simulink model "TypeBp"  (R2014a)
settings: Solver=ode45  StartTime=0.0  StopTime=10.0  RelTol=1e-3
values from neighbouring files (symbols this model uses):
  Act_Mat_BF = [     1,0,0,0,0,0;      0,1,0,0,0,0;      0,0,1,0,0,0;      0,0,0,1,0,0;      dv_BF,0,0,0,1,0;      0,0,0,0,0,1]    [param_PR3_noctr.m]
  Act_Mat_BR = [     1,0,0,0,0,0;      0,1,0,0,0,0;      0,0,1,0,0,0;      0,0,0,1,0,0;      dv_BR,0,0,0,1,0;      0,0,0,0,0,1]    [param_PR3_noctr.m]
  Act_Mat_IM = [     1,0,0,0,0,0;      0,1,0,0,0,0;      0,0,1,0,0,0;      0,0,0,1,0,0;      0,0,0,0,1,0;      0,0,0,0,0,1]    [param_PR3_noctr.m]
  Act_Mat_IR = [     1,0,0,0,0,0;      0,1,0,0,0,0;      0,0,1,0,0,0;      0,0,0,1,0,0;      0,0,0,0,1,0;      0,0,0,0,0,1]    [param_PR3_noctr.m]
  Act_Mat_RM = [     1,0,0,0,0,0;      0,1,0,0,0,0;      0,0,1,0,0,0;      0,0,0,1,0,0;      0,0,0,0,1,0;      0,0,0,0,0,1]    [param_PR3_noctr.m]
  Act_Mat_TM = [     1,0,0,0,0,0;      0,1,0,0,0,0;      0,0,1,0,0,0;      0,0,0,1,0,0;      0,0,0,0,1,0;      0,0,0,0,0,1]    [param_PR3_noctr.m]
  gain_act_LBF = 32.9296747504    [param_PR3_noctr.m]
  gain_act_LIM = 14.4730076835    [param_PR3_noctr.m]
  gain_act_LTM = 169.1045    [param_PR3_noctr.m]
  gain_act_PBF = 8.64557055148    [param_PR3_noctr.m]
  gain_act_PIM = 1.56040613295    [param_PR3_noctr.m]
  gain_act_PTM = 1.2097    [param_PR3_noctr.m]
  gain_act_RBF = 8.64557055148    [param_PR3_noctr.m]
  gain_act_RIM = 1.56632872419    [param_PR3_noctr.m]
  gain_act_TBF = 32.9154009359    [param_PR3_noctr.m]
  gain_act_TIM = 14.4745237388    [param_PR3_noctr.m]
  gain_act_VBF = 30.303030303    [param_PR3_noctr.m]
  gain_act_VF1 = 30.303030303    [param_PR3_noctr.m]
  gain_act_VF2 = 19.4037631453    [param_PR3_noctr.m]
  gain_act_VIM = 19.4037631453    [param_PR3_noctr.m]
  gain_act_YBF = 1.63692651118    [param_PR3_noctr.m]
  gain_act_YIM = 0.6169784052    [param_PR3_noctr.m]
  gain_act_YTM = 2.6742    [param_PR3_noctr.m]
  gain_global_LIM = 0    [param_PR3_noctr.m]
  gain_global_LTM = 0    [param_PR3_noctr.m]
  gain_LBF = 0    [param_PR3_noctr.m]
  gain_LIM = 0    [param_PR3_noctr.m]
  gain_oplev_LTM = 0    [param_PR3_noctr.m]
  gain_oplev_PIM = 0    [param_PR3_noctr.m]
  gain_oplev_PTM = 0    [param_PR3_noctr.m]
  gain_oplev_YIM = 0    [param_PR3_noctr.m]
  gain_oplev_YTM = 0    [param_PR3_noctr.m]
  gain_PBF = 0    [param_PR3_noctr.m]
  gain_PIM = 0    [param_PR3_noctr.m]
  gain_RBF = 0    [param_PR3_noctr.m]
  gain_RIM = 0    [param_PR3_noctr.m]
  gain_TBF = 0    [param_PR3_noctr.m]
  gain_TIM = 0    [param_PR3_noctr.m]
  gain_VBF = 0    [param_PR3_noctr.m]
  gain_VF1 = 0    [param_PR3_noctr.m]
  gain_VF2 = 0    [param_PR3_noctr.m]
  gain_VIM = 0    [param_PR3_noctr.m]
  gain_YBF = 0    [param_PR3_noctr.m]
  gain_YIM = 0    [param_PR3_noctr.m]
  Sens_Mat_OL = [     1,0,0,0,0,0;      0,1,0,0,0,0;      0,0,1,0,0,0;      0,0,0,1,0,0;      0,0,0,0,1,0;      0,0,0,0,0,1]    [param_PR3_noctr.m]
undefined symbols (not defined in the file or in its folder): sys1
libraries: cstblocks x21, simulink x3
settings Model: Creator=TAMA Project  LastModifiedBy=FYY
settings DataIOCC: SignalLoggingSaveFormat=ModelDataLogs
settings OptimizationCC: ExpressionDepthLimit=2147483647
settings DebuggingCC: UnderspecifiedInitializationDetection=Classic  FcnCallInpInsideContextMsg=UseLocalSettings  StateNameClashWarn=warning
settings GRTTargetCC: CombineOutputUpdateFcns=off  GRTInterface=on

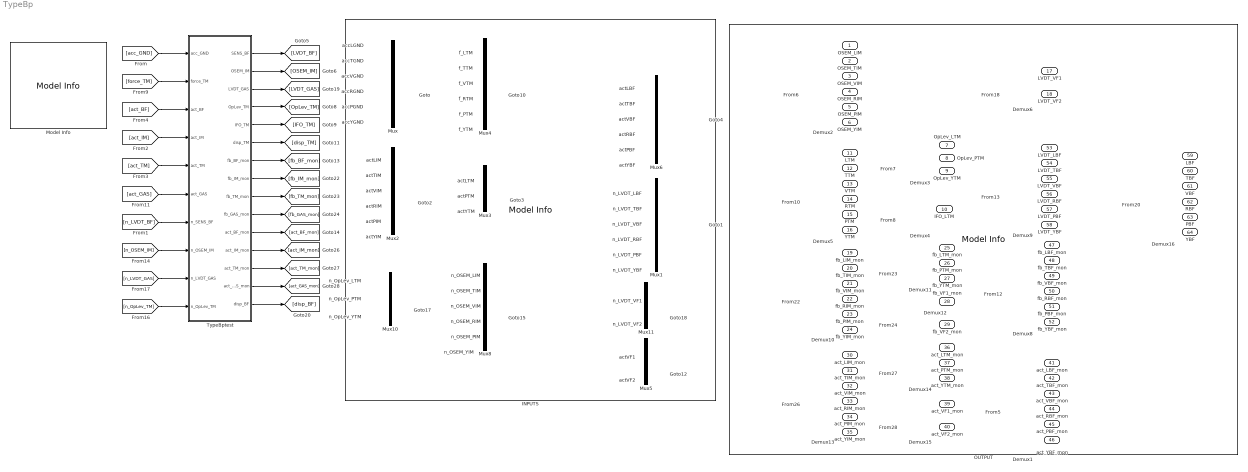
== system TypeBp ==
  accLGND : Inport
  accTGND : Inport  Port=2
  accVGND : Inport  Port=3
  accRGND : Inport  Port=4
  accPGND : Inport  Port=5
  accYGND : Inport  Port=6
  actLIM : Inport  Port=7
  actTIM : Inport  Port=8
  actVIM : Inport  Port=9
  actRIM : Inport  Port=10
  actPIM : Inport  Port=11
  actYIM : Inport  Port=12
  actLTM : Inport  Port=13
  actPTM : Inport  Port=14
  actYTM : Inport  Port=15
  f_LTM : Inport  Port=16
  f_TTM : Inport  Port=17
  f_VTM : Inport  Port=18
  f_RTM : Inport  Port=19
  f_PTM : Inport  Port=20
  f_YTM : Inport  Port=21
  actVF1 : Inport  Port=22
  actVF2 : Inport  Port=23
  n_OSEM_LIM : Inport  Port=24
  n_OSEM_TIM : Inport  Port=25
  n_OSEM_VIM : Inport  Port=26
  n_OSEM_RIM : Inport  Port=27
  n_OSEM_PIM : Inport  Port=28
  n_OSEM_YIM : Inport  Port=29
  n_OpLev_LTM : Inport  Port=30
  n_OpLev_PTM : Inport  Port=31
  n_OpLev_YTM : Inport  Port=32
  n_LVDT_VF1 : Inport  Port=33
  n_LVDT_VF2 : Inport  Port=34
  n_LVDT_LBF : Inport  Port=35
  n_LVDT_TBF : Inport  Port=36
  n_LVDT_VBF : Inport  Port=37
  n_LVDT_RBF : Inport  Port=38
  n_LVDT_PBF : Inport  Port=39
  n_LVDT_YBF : Inport  Port=40
  actLBF : Inport  Port=41
  actTBF : Inport  Port=42
  actVBF : Inport  Port=43
  actRBF : Inport  Port=44
  actPBF : Inport  Port=45
  actYBF : Inport  Port=46
  Demux{1..2,5,8..10,13,16} (8 alike) : Demux  Outputs=6
  Demux11 : Demux  Outputs=3
  Demux12 : Demux  Outputs=2
  Demux14 : Demux  Outputs=3
  Demux15 : Demux  Outputs=2
  Demux3 : Demux  Outputs=3
  Demux4 : Demux  Outputs=1
  Demux6 : Demux  Outputs=2
  INPUTS : simulink/Model-Wide Utilities/Model Info  InitialBlockCM=なし  Frame=on  DisplayStringWithTags=_  HorizontalTextAlignment=Left  LeftAlignmentValue=0.02  SourceBlockDiagram=typeBp161115simctrl_LengthOL  TagMaxNumber=20
  Model Info : simulink/Model-Wide Utilities/Model Info  InitialBlockCM=なし  Frame=on  DisplayStringWithTags=|  HorizontalTextAlignment=Left  LeftAlignmentValue=0.02  SourceBlockDiagram=typeBp161115simctrl_LengthOL  TagMaxNumber=20
      | [MODEL INFORMATION]
      | 
      | ModelName: %<ModelName>
      | LastUpdate : %<LastModificationDate>
      | 
      | TypeBp control model
  Mux{,1..2,4,6,8} (6 alike) : Mux  Inputs=6
  Mux10 : Mux  Inputs=3
  Mux11 : Mux  Inputs=2
  Mux3 : Mux  Inputs=3
  Mux5 : Mux  Inputs=2
  OUTPUT : simulink/Model-Wide Utilities/Model Info  InitialBlockCM=なし  Frame=on  DisplayStringWithTags=_  HorizontalTextAlignment=Left  LeftAlignmentValue=0.02  SourceBlockDiagram=typeBp161115simctrl_LengthOL  TagMaxNumber=20
  TypeBptest : Subsystem
  OSEM_LIM : Outport
  OSEM_TIM : Outport  Port=2
  OSEM_VIM : Outport  Port=3
  OSEM_RIM : Outport  Port=4
  OSEM_PIM : Outport  Port=5
  OSEM_YIM : Outport  Port=6
  OpLev_LTM : Outport  Port=7
  OpLev_PTM : Outport  Port=8
  OpLev_YTM : Outport  Port=9
  IFO_LTM : Outport  Port=10
  LTM : Outport  Port=11
  TTM : Outport  Port=12
  VTM : Outport  Port=13
  RTM : Outport  Port=14
  PTM : Outport  Port=15
  YTM : Outport  Port=16
  LVDT_VF1 : Outport  Port=17
  LVDT_VF2 : Outport  Port=18
  fb_LIM_mon : Outport  Port=19
  fb_TIM_mon : Outport  Port=20
  fb_VIM_mon : Outport  Port=21
  fb_RIM_mon : Outport  Port=22
  fb_PIM_mon : Outport  Port=23
  fb_YIM_mon : Outport  Port=24
  fb_LTM_mon : Outport  Port=25
  fb_PTM_mon : Outport  Port=26
  fb_YTM_mon : Outport  Port=27
  fb_VF1_mon : Outport  Port=28
  fb_VF2_mon : Outport  Port=29
  act_LIM_mon : Outport  Port=30
  act_TIM_mon : Outport  Port=31
  act_VIM_mon : Outport  Port=32
  act_RIM_mon : Outport  Port=33
  act_PIM_mon : Outport  Port=34
  act_YIM_mon : Outport  Port=35
  act_LTM_mon : Outport  Port=36
  act_PTM_mon : Outport  Port=37
  act_YTM_mon : Outport  Port=38
  act_VF1_mon : Outport  Port=39
  act_VF2_mon : Outport  Port=40
  act_LBF_mon : Outport  Port=41
  act_TBF_mon : Outport  Port=42
  act_VBF_mon : Outport  Port=43
  act_RBF_mon : Outport  Port=44
  act_PBF_mon : Outport  Port=45
  act_YBF_mon : Outport  Port=46
  fb_LBF_mon : Outport  Port=47
  fb_TBF_mon : Outport  Port=48
  fb_VBF_mon : Outport  Port=49
  fb_RBF_mon : Outport  Port=50
  fb_PBF_mon : Outport  Port=51
  fb_YBF_mon : Outport  Port=52
  LVDT_LBF : Outport  Port=53
  LVDT_TBF : Outport  Port=54
  LVDT_VBF : Outport  Port=55
  LVDT_RBF : Outport  Port=56
  LVDT_PBF : Outport  Port=57
  LVDT_YBF : Outport  Port=58
  LBF : Outport  Port=59
  TBF : Outport  Port=60
  VBF : Outport  Port=61
  RBF : Outport  Port=62
  PBF : Outport  Port=63
  YBF : Outport  Port=64
  wires:
  accLGND/1 -> Mux/1
  accTGND/1 -> Mux/2
  accVGND/1 -> Mux/3
  accRGND/1 -> Mux/4
  accPGND/1 -> Mux/5
  accYGND/1 -> Mux/6
  Mux/1 -> [acc_GND]
  actLIM/1 -> Mux2/1
  actTIM/1 -> Mux2/2
  actVIM/1 -> Mux2/3
  actRIM/1 -> Mux2/4
  actPIM/1 -> Mux2/5
  actYIM/1 -> Mux2/6
  Mux2/1 -> [act_IM]
  actLTM/1 -> Mux3/1
  actPTM/1 -> Mux3/2
  actYTM/1 -> Mux3/3
  Mux3/1 -> [act_TM]
  [OSEM_IM] -> Demux2/1
  Demux2/1 -> OSEM_LIM/1
  Demux2/2 -> OSEM_TIM/1
  Demux2/3 -> OSEM_VIM/1
  Demux2/4 -> OSEM_RIM/1
  Demux2/5 -> OSEM_PIM/1
  Demux2/6 -> OSEM_YIM/1
  [IFO_TM] -> Demux4/1
  Demux4/1 -> IFO_LTM/1
  f_LTM/1 -> Mux4/1
  f_TTM/1 -> Mux4/2
  f_VTM/1 -> Mux4/3
  Mux4/1 -> [force_TM]
  f_YTM/1 -> Mux4/6
  f_PTM/1 -> Mux4/5
  f_RTM/1 -> Mux4/4
  [disp_TM] -> Demux5/1
  Demux5/1 -> LTM/1
  Demux5/2 -> TTM/1
  Demux5/3 -> VTM/1
  Demux5/4 -> RTM/1
  Demux5/5 -> PTM/1
  Demux5/6 -> YTM/1
  actVF2/1 -> Mux5/2
  Mux5/1 -> [act_GAS]
  n_OSEM_LIM/1 -> Mux8/1
  n_OSEM_TIM/1 -> Mux8/2
  n_OSEM_VIM/1 -> Mux8/3
  n_OSEM_RIM/1 -> Mux8/4
  n_OSEM_PIM/1 -> Mux8/5
  n_OSEM_YIM/1 -> Mux8/6
  Mux8/1 -> [n_OSEM_IM]
  Mux10/1 -> [n_OpLev_TM]
  n_LVDT_VF2/1 -> Mux11/2
  Mux11/1 -> [n_LVDT_GAS]
  [LVDT_GAS] -> Demux6/1
  n_LVDT_VF1/1 -> Mux11/1
  Demux6/1 -> LVDT_VF1/1
  Demux6/2 -> LVDT_VF2/1
  actVF1/1 -> Mux5/1
  [fb_IM_mon] -> Demux10/1
  Demux10/1 -> fb_LIM_mon/1
  Demux10/2 -> fb_TIM_mon/1
  Demux10/3 -> fb_VIM_mon/1
  Demux10/4 -> fb_RIM_mon/1
  Demux10/5 -> fb_PIM_mon/1
  Demux10/6 -> fb_YIM_mon/1
  [fb_TM_mon] -> Demux11/1
  Demux11/1 -> fb_LTM_mon/1
  Demux11/2 -> fb_PTM_mon/1
  Demux11/3 -> fb_YTM_mon/1
  [fb_GAS_mon] -> Demux12/1
  Demux12/1 -> fb_VF1_mon/1
  Demux12/2 -> fb_VF2_mon/1
  [act_IM_mon] -> Demux13/1
  Demux13/1 -> act_LIM_mon/1
  Demux13/2 -> act_TIM_mon/1
  Demux13/3 -> act_VIM_mon/1
  Demux13/4 -> act_RIM_mon/1
  Demux13/5 -> act_PIM_mon/1
  Demux13/6 -> act_YIM_mon/1
  [act_TM_mon] -> Demux14/1
  Demux14/1 -> act_LTM_mon/1
  Demux14/2 -> act_PTM_mon/1
  Demux14/3 -> act_YTM_mon/1
  [act_GAS_mon] -> Demux15/1
  Demux15/1 -> act_VF1_mon/1
  Demux15/2 -> act_VF2_mon/1
  n_LVDT_TBF/1 -> Mux1/2
  Mux1/1 -> [n_LVDT_BF]
  n_LVDT_LBF/1 -> Mux1/1
  n_LVDT_VBF/1 -> Mux1/3
  actTBF/1 -> Mux6/2
  Mux6/1 -> [act_BF]
  actLBF/1 -> Mux6/1
  actVBF/1 -> Mux6/3
  [act_BF_mon] -> Demux1/1
  Demux1/1 -> act_LBF_mon/1
  Demux1/2 -> act_TBF_mon/1
  Demux1/3 -> act_VBF_mon/1
  [fb_BF_mon] -> Demux8/1
  Demux8/1 -> fb_LBF_mon/1
  Demux8/2 -> fb_TBF_mon/1
  Demux8/3 -> fb_VBF_mon/1
  [LVDT_BF] -> Demux9/1
  Demux9/1 -> LVDT_LBF/1
  Demux9/2 -> LVDT_TBF/1
  Demux9/3 -> LVDT_VBF/1
  [acc_GND] -> TypeBptest/1(acc_GND)
  [force_TM] -> TypeBptest/2(force_TM)
  [act_BF] -> TypeBptest/3(act_BF)
  [act_IM] -> TypeBptest/4(act_IM)
  [act_TM] -> TypeBptest/5(act_TM)
  [act_GAS] -> TypeBptest/6(act_GAS)
  [n_LVDT_BF] -> TypeBptest/7(n_SENS_BF)
  [n_OSEM_IM] -> TypeBptest/8(n_OSEM_IM)
  [n_LVDT_GAS] -> TypeBptest/9(n_LVDT_GAS)
  [n_OpLev_TM] -> TypeBptest/10(n_OpLev_TM)
  TypeBptest/1(SENS_BF) -> [LVDT_BF]
  TypeBptest/2(OSEM_IM) -> [OSEM_IM]
  TypeBptest/3(LVDT_GAS) -> [LVDT_GAS]
  TypeBptest/4(OpLev_TM) -> [OpLev_TM]
  TypeBptest/5(IFO_TM) -> [IFO_TM]
  TypeBptest/6(disp_TM) -> [disp_TM]
  TypeBptest/7(fb_BF_mon) -> [fb_BF_mon]
  TypeBptest/8(fb_IM_mon) -> [fb_IM_mon]
  TypeBptest/9(fb_TM_mon) -> [fb_TM_mon]
  TypeBptest/10(fb_GAS_mon) -> [fb_GAS_mon]
  TypeBptest/12(act_IM_mon) -> [act_IM_mon]
  TypeBptest/14(act_GAS_mon) -> [act_GAS_mon]
  actRBF/1 -> Mux6/4
  actPBF/1 -> Mux6/5
  actYBF/1 -> Mux6/6
  n_LVDT_RBF/1 -> Mux1/4
  n_LVDT_PBF/1 -> Mux1/5
  n_LVDT_YBF/1 -> Mux1/6
  Demux9/4 -> LVDT_RBF/1
  Demux9/5 -> LVDT_PBF/1
  Demux9/6 -> LVDT_YBF/1
  Demux8/4 -> fb_RBF_mon/1
  Demux8/5 -> fb_PBF_mon/1
  Demux8/6 -> fb_YBF_mon/1
  Demux1/4 -> act_RBF_mon/1
  Demux1/5 -> act_PBF_mon/1
  Demux1/6 -> act_YBF_mon/1
  TypeBptest/15(disp_BF) -> [disp_BF]
  [disp_BF] -> Demux16/1
  Demux16/1 -> LBF/1
  Demux16/2 -> TBF/1
  Demux16/3 -> VBF/1
  Demux16/4 -> RBF/1
  Demux16/5 -> PBF/1
  Demux16/6 -> YBF/1
  TypeBptest/11(act_BF_mon) -> [act_BF_mon]
  TypeBptest/13(act_TM_mon) -> [act_TM_mon]
  n_OpLev_PTM/1 -> Mux10/2
  n_OpLev_LTM/1 -> Mux10/1
  n_OpLev_YTM/1 -> Mux10/3
  Demux3/2 -> OpLev_PTM/1
  Demux3/3 -> OpLev_YTM/1
  Demux3/1 -> OpLev_LTM/1
  [OpLev_TM] -> Demux3/1

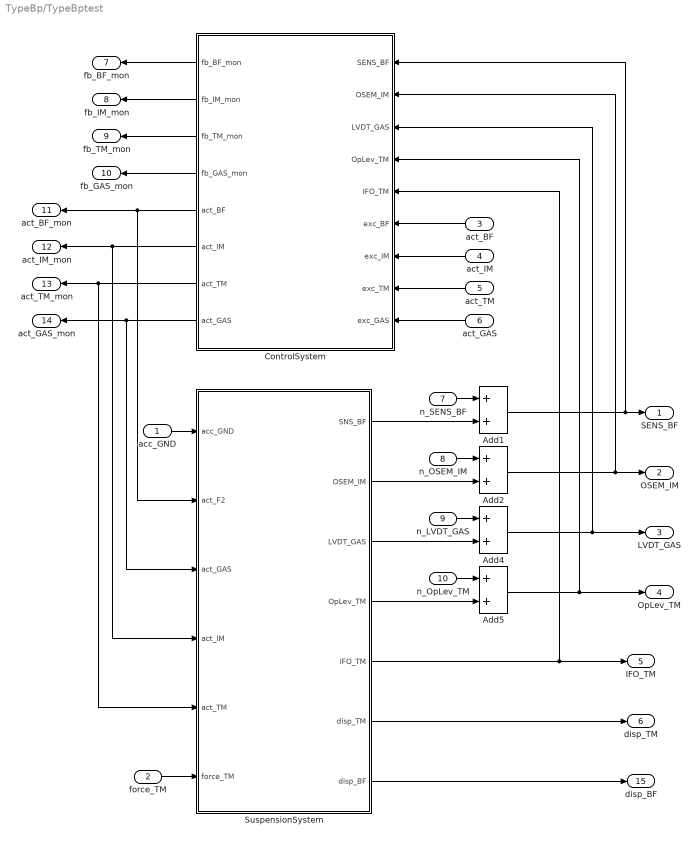
== system TypeBp/TypeBptest ==
  acc_GND : Inport
  force_TM : Inport  Port=2
  act_BF : Inport  Port=3
  act_IM : Inport  Port=4
  act_TM : Inport  Port=5
  act_GAS : Inport  Port=6
  n_SENS_BF : Inport  Port=7
  n_OSEM_IM : Inport  Port=8
  n_LVDT_GAS : Inport  Port=9
  n_OpLev_TM : Inport  Port=10
  Add{1..2,4..5} (4 alike) : Sum
  ControlSystem : Subsystem
  SuspensionSystem : Subsystem
  SENS_BF : Outport
  OSEM_IM : Outport  Port=2
  LVDT_GAS : Outport  Port=3
  OpLev_TM : Outport  Port=4
  IFO_TM : Outport  Port=5
  disp_TM : Outport  Port=6
  fb_BF_mon : Outport  Port=7
  fb_IM_mon : Outport  Port=8
  fb_TM_mon : Outport  Port=9
  fb_GAS_mon : Outport  Port=10
  act_BF_mon : Outport  Port=11
  act_IM_mon : Outport  Port=12
  act_TM_mon : Outport  Port=13
  act_GAS_mon : Outport  Port=14
  disp_BF : Outport  Port=15
  wires:
  acc_GND/1 -> SuspensionSystem/1(acc_GND)
  force_TM/1 -> SuspensionSystem/6(force_TM)
  SuspensionSystem/6(disp_TM) -> disp_TM/1
  SuspensionSystem/2(OSEM_IM) -> Add2/2
  n_OSEM_IM/1 -> Add2/1
  SuspensionSystem/5(IFO_TM) -> IFO_TM/1, ControlSystem/5(IFO_TM)
  Add2/1 -> ControlSystem/2(OSEM_IM), OSEM_IM/1
  n_LVDT_GAS/1 -> Add4/1
  SuspensionSystem/3(LVDT_GAS) -> Add4/2
  n_OpLev_TM/1 -> Add5/1
  SuspensionSystem/4(OpLev_TM) -> Add5/2
  Add4/1 -> ControlSystem/3(LVDT_GAS), LVDT_GAS/1
  Add5/1 -> ControlSystem/4(OpLev_TM), OpLev_TM/1
  Add1/1 -> ControlSystem/1(SENS_BF), SENS_BF/1
  SuspensionSystem/1(SNS_BF) -> Add1/2
  n_SENS_BF/1 -> Add1/1
  act_BF/1 -> ControlSystem/6(exc_BF)
  act_IM/1 -> ControlSystem/7(exc_IM)
  act_TM/1 -> ControlSystem/8(exc_TM)
  act_GAS/1 -> ControlSystem/9(exc_GAS)
  ControlSystem/1(fb_BF_mon) -> fb_BF_mon/1
  ControlSystem/2(fb_IM_mon) -> fb_IM_mon/1
  ControlSystem/3(fb_TM_mon) -> fb_TM_mon/1
  ControlSystem/4(fb_GAS_mon) -> fb_GAS_mon/1
  ControlSystem/5(act_BF) -> SuspensionSystem/2(act_F2), act_BF_mon/1
  ControlSystem/7(act_TM) -> SuspensionSystem/5(act_TM), act_TM_mon/1
  ControlSystem/8(act_GAS) -> SuspensionSystem/3(act_GAS), act_GAS_mon/1
  ControlSystem/6(act_IM) -> SuspensionSystem/4(act_IM), act_IM_mon/1
  SuspensionSystem/7(disp_BF) -> disp_BF/1

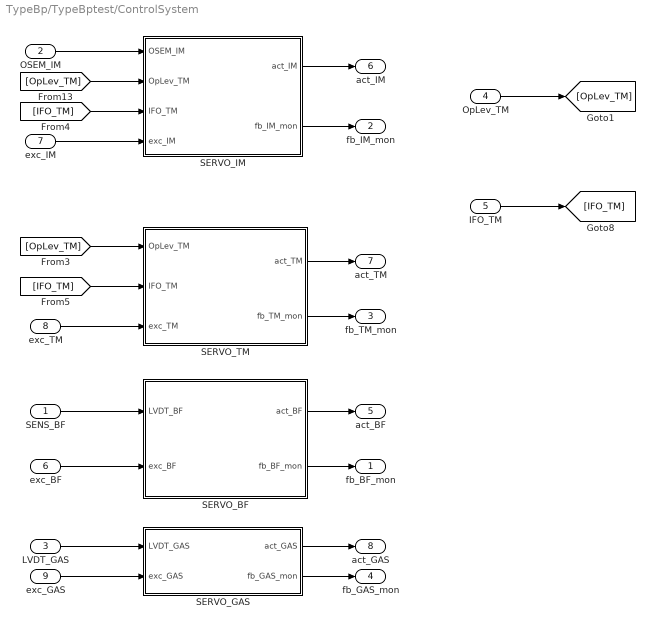
== system TypeBp/TypeBptest/ControlSystem ==
  SENS_BF : Inport
  OSEM_IM : Inport  Port=2
  LVDT_GAS : Inport  Port=3
  OpLev_TM : Inport  Port=4
  IFO_TM : Inport  Port=5
  exc_BF : Inport  Port=6
  exc_IM : Inport  Port=7
  exc_TM : Inport  Port=8
  exc_GAS : Inport  Port=9
  SERVO_BF : Subsystem
  SERVO_GAS : Subsystem
  SERVO_IM : Subsystem
  SERVO_TM : Subsystem
  fb_BF_mon : Outport
  fb_IM_mon : Outport  Port=2
  fb_TM_mon : Outport  Port=3
  fb_GAS_mon : Outport  Port=4
  act_BF : Outport  Port=5
  act_IM : Outport  Port=6
  act_TM : Outport  Port=7
  act_GAS : Outport  Port=8
  wires:
  IFO_TM/1 -> [IFO_TM]
  OpLev_TM/1 -> [OpLev_TM]
  SERVO_IM/1(act_IM) -> act_IM/1
  OSEM_IM/1 -> SERVO_IM/1(OSEM_IM)
  SERVO_TM/1(act_TM) -> act_TM/1
  [OpLev_TM] -> SERVO_IM/2(OpLev_TM)
  [OpLev_TM] -> SERVO_TM/1(OpLev_TM)
  [IFO_TM] -> SERVO_IM/3(IFO_TM)
  [IFO_TM] -> SERVO_TM/2(IFO_TM)
  exc_IM/1 -> SERVO_IM/4(exc_IM)
  exc_TM/1 -> SERVO_TM/3(exc_TM)
  SERVO_IM/2(fb_IM_mon) -> fb_IM_mon/1
  SERVO_TM/2(fb_TM_mon) -> fb_TM_mon/1
  exc_GAS/1 -> SERVO_GAS/2(exc_GAS)
  SERVO_GAS/2(fb_GAS_mon) -> fb_GAS_mon/1
  LVDT_GAS/1 -> SERVO_GAS/1(LVDT_GAS)
  SERVO_GAS/1(act_GAS) -> act_GAS/1
  SENS_BF/1 -> SERVO_BF/1(LVDT_BF)
  SERVO_BF/1(act_BF) -> act_BF/1
  exc_BF/1 -> SERVO_BF/2(exc_BF)
  SERVO_BF/2(fb_BF_mon) -> fb_BF_mon/1

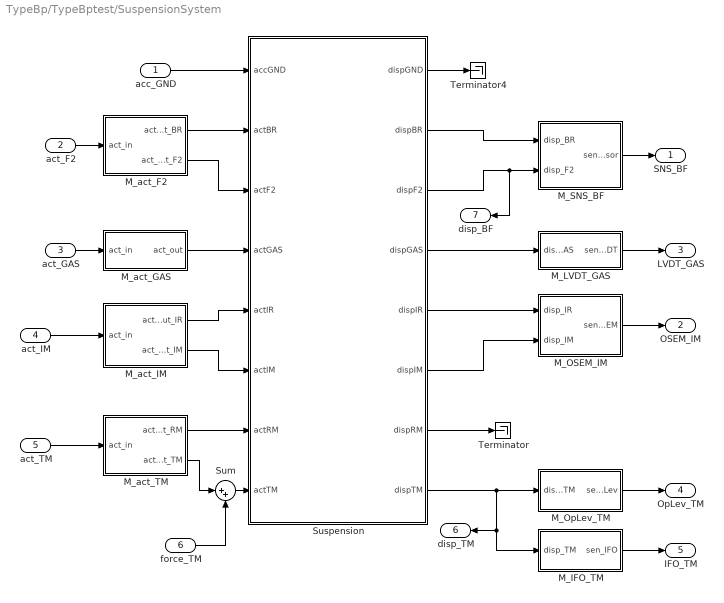
== system TypeBp/TypeBptest/SuspensionSystem ==
  acc_GND : Inport
  act_F2 : Inport  Port=2
  act_GAS : Inport  Port=3
  act_IM : Inport  Port=4
  act_TM : Inport  Port=5
  force_TM : Inport  Port=6
  M_IFO_TM : Subsystem
  M_LVDT_GAS : Subsystem
  M_OSEM_IM : Subsystem
  M_OpLev_TM : Subsystem
  M_SNS_BF : Subsystem
  M_act_F2 : Subsystem
  M_act_GAS : Subsystem
  M_act_IM : Subsystem
  M_act_TM : Subsystem
  Sum : Sum  Inputs=|++
  Suspension : Subsystem
  Terminator : Terminator
  Terminator4 : Terminator
  SNS_BF : Outport
  OSEM_IM : Outport  Port=2
  LVDT_GAS : Outport  Port=3
  OpLev_TM : Outport  Port=4
  IFO_TM : Outport  Port=5
  disp_TM : Outport  Port=6
  disp_BF : Outport  Port=7
  wires:
  act_IM/1 -> M_act_IM/1(act_in)
  act_TM/1 -> M_act_TM/1(act_in)
  act_GAS/1 -> M_act_GAS/1(act_in)
  M_OSEM_IM/1(sen_OSEM) -> OSEM_IM/1
  M_LVDT_GAS/1(sen_LVDT) -> LVDT_GAS/1
  M_IFO_TM/1(sen_IFO) -> IFO_TM/1
  M_OpLev_TM/1(sen_OpLev) -> OpLev_TM/1
  act_F2/1 -> M_act_F2/1(act_in)
  acc_GND/1 -> Suspension/1(accGND)
  M_act_F2/1(act_out_BR) -> Suspension/2(actBR)
  M_act_F2/2(act_out_F2) -> Suspension/3(actF2)
  M_act_GAS/1(act_out) -> Suspension/4(actGAS)
  M_act_IM/1(act_out_IR) -> Suspension/5(actIR)
  M_act_IM/2(act_out_IM) -> Suspension/6(actIM)
  M_act_TM/1(act_out_RM) -> Suspension/7(actRM)
  M_act_TM/2(act_out_TM) -> Sum/1
  force_TM/1 -> Sum/2
  Sum/1 -> Suspension/8(actTM)
  M_SNS_BF/1(sen_F2sensor) -> SNS_BF/1
  Suspension/2(dispBR) -> M_SNS_BF/1(disp_BR)
  Suspension/3(dispF2) -> disp_BF/1, M_SNS_BF/2(disp_F2)
  Suspension/1(dispGND) -> Terminator4/1
  Suspension/4(dispGAS) -> M_LVDT_GAS/1(disp_GAS)
  Suspension/5(dispIR) -> M_OSEM_IM/1(disp_IR)
  Suspension/6(dispIM) -> M_OSEM_IM/2(disp_IM)
  Suspension/8(dispTM) -> M_IFO_TM/1(disp_TM), disp_TM/1, M_OpLev_TM/1(disp_TM)
  Suspension/7(dispRM) -> Terminator/1

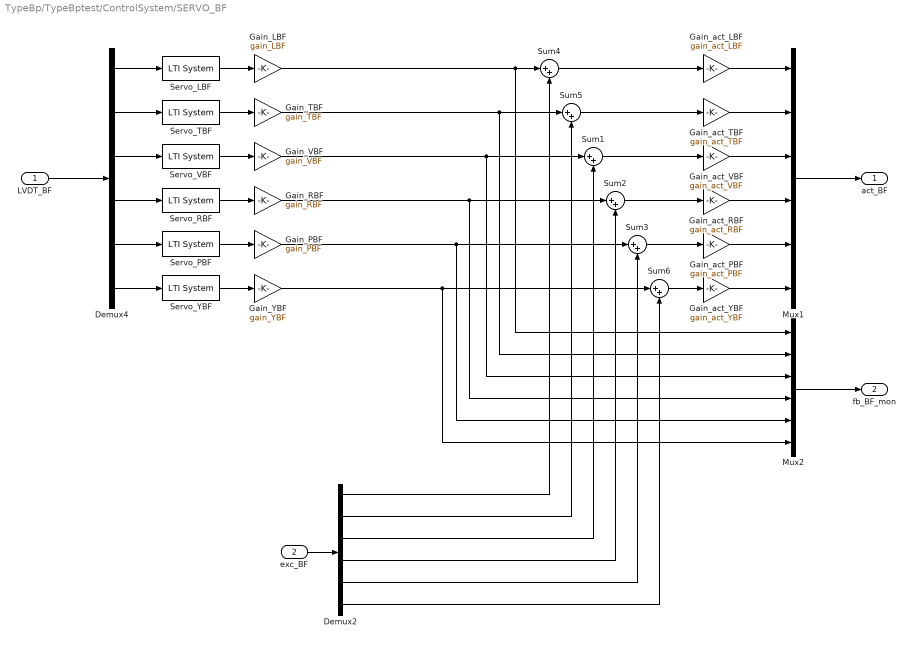
== system TypeBp/TypeBptest/ControlSystem/SERVO_BF ==
  LVDT_BF : Inport
  exc_BF : Inport  Port=2
  Demux2 : Demux  Outputs=6
  Demux4 : Demux  Outputs=6
  Gain_LBF : Gain  Gain=gain_LBF
  Gain_PBF : Gain  Gain=gain_PBF
  Gain_RBF : Gain  Gain=gain_RBF
  Gain_TBF : Gain  Gain=gain_TBF
  Gain_VBF : Gain  Gain=gain_VBF
  Gain_YBF : Gain  Gain=gain_YBF
  Gain_act_LBF : Gain  Gain=gain_act_LBF
  Gain_act_PBF : Gain  Gain=gain_act_PBF
  Gain_act_RBF : Gain  Gain=gain_act_RBF
  Gain_act_TBF : Gain  Gain=gain_act_TBF
  Gain_act_VBF : Gain  Gain=gain_act_VBF
  Gain_act_YBF : Gain  Gain=gain_act_YBF
  Mux1 : Mux  Inputs=6
  Mux2 : Mux  Inputs=6
  Servo_LBF : cstblocks/LTI System  sys=servo_LBF  IC=[]
  Servo_PBF : cstblocks/LTI System  sys=servo_PBF  IC=[]
  Servo_RBF : cstblocks/LTI System  sys=servo_RBF  IC=[]
  Servo_TBF : cstblocks/LTI System  sys=servo_TBF  IC=[]
  Servo_VBF : cstblocks/LTI System  sys=servo_VBF  IC=[]
  Servo_YBF : cstblocks/LTI System  sys=servo_YBF  IC=[]
  Sum{1..6} (6 alike) : Sum  Inputs=|++
  act_BF : Outport
  fb_BF_mon : Outport  Port=2
  wires:
  Demux4/1 -> Servo_LBF/1
  Demux4/2 -> Servo_TBF/1
  Servo_LBF/1 -> Gain_LBF/1
  Servo_TBF/1 -> Gain_TBF/1
  LVDT_BF/1 -> Demux4/1
  Mux1/1 -> act_BF/1
  Gain_act_LBF/1 -> Mux1/1
  Gain_act_TBF/1 -> Mux1/2
  Gain_LBF/1 -> Mux2/1, Sum4/1
  Sum4/1 -> Gain_act_LBF/1
  Gain_TBF/1 -> Mux2/2, Sum5/1
  Sum5/1 -> Gain_act_TBF/1
  exc_BF/1 -> Demux2/1
  Mux2/1 -> fb_BF_mon/1
  Demux4/3 -> Servo_VBF/1
  Servo_VBF/1 -> Gain_VBF/1
  Gain_act_VBF/1 -> Mux1/3
  Sum1/1 -> Gain_act_VBF/1
  Gain_VBF/1 -> Mux2/3, Sum1/1
  Demux2/1 -> Sum4/2
  Demux2/2 -> Sum5/2
  Demux2/3 -> Sum1/2
  Demux4/4 -> Servo_RBF/1
  Servo_RBF/1 -> Gain_RBF/1
  Gain_act_RBF/1 -> Mux1/4
  Gain_RBF/1 -> Mux2/4, Sum2/1
  Sum2/1 -> Gain_act_RBF/1
  Demux4/5 -> Servo_PBF/1
  Servo_PBF/1 -> Gain_PBF/1
  Gain_act_PBF/1 -> Mux1/5
  Gain_PBF/1 -> Mux2/5, Sum3/1
  Sum3/1 -> Gain_act_PBF/1
  Demux4/6 -> Servo_YBF/1
  Servo_YBF/1 -> Gain_YBF/1
  Gain_act_YBF/1 -> Mux1/6
  Gain_YBF/1 -> Mux2/6, Sum6/1
  Sum6/1 -> Gain_act_YBF/1
  Demux2/4 -> Sum2/2
  Demux2/5 -> Sum3/2
  Demux2/6 -> Sum6/2

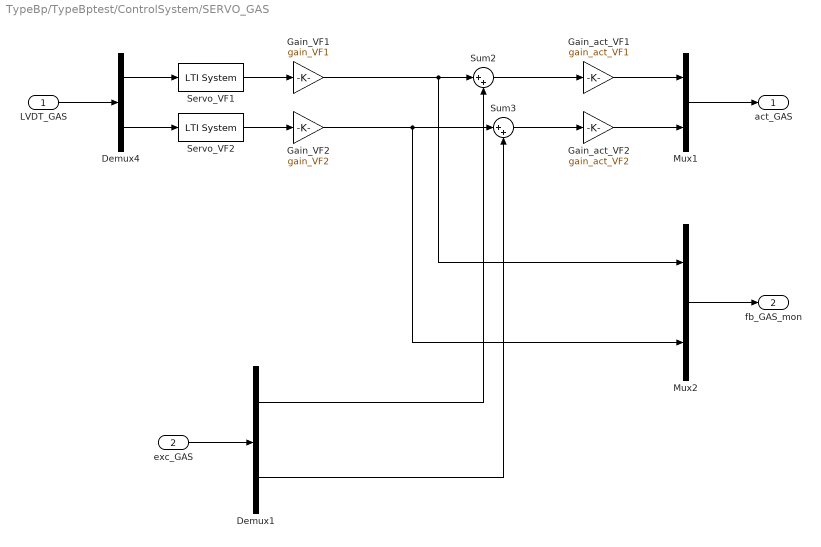
== system TypeBp/TypeBptest/ControlSystem/SERVO_GAS ==
  LVDT_GAS : Inport
  exc_GAS : Inport  Port=2
  Demux1 : Demux  Outputs=2
  Demux4 : Demux  Outputs=2
  Gain_VF1 : Gain  Gain=gain_VF1
  Gain_VF2 : Gain  Gain=gain_VF2
  Gain_act_VF1 : Gain  Gain=gain_act_VF1
  Gain_act_VF2 : Gain  Gain=gain_act_VF2
  Mux1 : Mux  Inputs=2
  Mux2 : Mux  Inputs=2
  Servo_VF1 : cstblocks/LTI System  sys=servo_VF1  IC=[]
  Servo_VF2 : cstblocks/LTI System  sys=servo_VF2  IC=[]
  Sum2 : Sum  Inputs=|++
  Sum3 : Sum  Inputs=|++
  act_GAS : Outport
  fb_GAS_mon : Outport  Port=2
  wires:
  Servo_VF1/1 -> Gain_VF1/1
  Servo_VF2/1 -> Gain_VF2/1
  LVDT_GAS/1 -> Demux4/1
  Mux1/1 -> act_GAS/1
  exc_GAS/1 -> Demux1/1
  Gain_VF1/1 -> Mux2/1, Sum2/1
  Sum2/1 -> Gain_act_VF1/1
  Gain_VF2/1 -> Mux2/2, Sum3/1
  Sum3/1 -> Gain_act_VF2/1
  Mux2/1 -> fb_GAS_mon/1
  Demux4/1 -> Servo_VF1/1
  Demux4/2 -> Servo_VF2/1
  Gain_act_VF1/1 -> Mux1/1
  Gain_act_VF2/1 -> Mux1/2
  Demux1/1 -> Sum2/2
  Demux1/2 -> Sum3/2

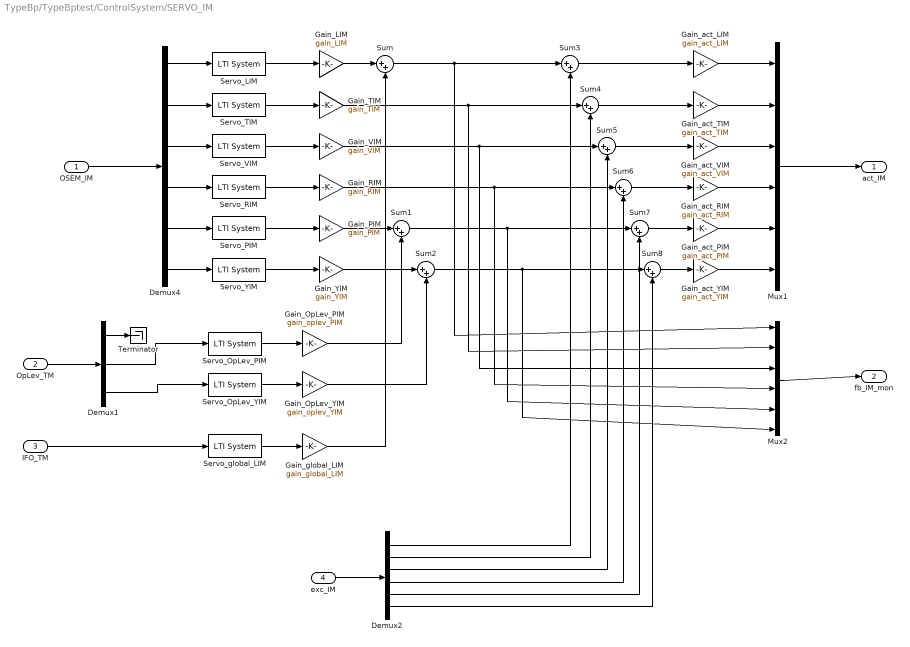
== system TypeBp/TypeBptest/ControlSystem/SERVO_IM ==
  OSEM_IM : Inport
  OpLev_TM : Inport  Port=2
  IFO_TM : Inport  Port=3
  exc_IM : Inport  Port=4
  Demux1 : Demux  Outputs=3
  Demux2 : Demux  Outputs=6
  Demux4 : Demux  Outputs=6
  Gain_LIM : Gain  Gain=gain_LIM
  Gain_OpLev_PIM : Gain  Gain=gain_oplev_PIM
  Gain_OpLev_YIM : Gain  Gain=gain_oplev_YIM
  Gain_PIM : Gain  Gain=gain_PIM
  Gain_RIM : Gain  Gain=gain_RIM
  Gain_TIM : Gain  Gain=gain_TIM
  Gain_VIM : Gain  Gain=gain_VIM
  Gain_YIM : Gain  Gain=gain_YIM
  Gain_act_LIM : Gain  Gain=gain_act_LIM
  Gain_act_PIM : Gain  Gain=gain_act_PIM
  Gain_act_RIM : Gain  Gain=gain_act_RIM
  Gain_act_TIM : Gain  Gain=gain_act_TIM
  Gain_act_VIM : Gain  Gain=gain_act_VIM
  Gain_act_YIM : Gain  Gain=gain_act_YIM
  Gain_global_LIM : Gain  Gain=gain_global_LIM
  Mux1 : Mux  Inputs=6
  Mux2 : Mux  Inputs=6
  Servo_LIM : cstblocks/LTI System  sys=servo_LIM  IC=[]
  Servo_OpLev_PIM : cstblocks/LTI System  sys=servo_oplev_PIM  IC=[]
  Servo_OpLev_YIM : cstblocks/LTI System  sys=servo_oplev_YIM  IC=[]
  Servo_PIM : cstblocks/LTI System  sys=servo_PIM  IC=[]
  Servo_RIM : cstblocks/LTI System  sys=servo_RIM  IC=[]
  Servo_TIM : cstblocks/LTI System  sys=servo_TIM  IC=[]
  Servo_VIM : cstblocks/LTI System  sys=servo_VIM  IC=[]
  Servo_YIM : cstblocks/LTI System  sys=servo_YIM  IC=[]
  Servo_global_LIM : cstblocks/LTI System  sys=servo_global_LIM  IC=[]
  Sum{,1..8} (9 alike) : Sum  Inputs=|++
  Terminator : Terminator
  act_IM : Outport
  fb_IM_mon : Outport  Port=2
  wires:
  Demux4/1 -> Servo_LIM/1
  Demux4/2 -> Servo_TIM/1
  Demux4/3 -> Servo_VIM/1
  Servo_LIM/1 -> Gain_LIM/1
  Servo_TIM/1 -> Gain_TIM/1
  Servo_VIM/1 -> Gain_VIM/1
  Mux1/1 -> act_IM/1
  Gain_act_LIM/1 -> Mux1/1
  Gain_act_TIM/1 -> Mux1/2
  Gain_act_VIM/1 -> Mux1/3
  OSEM_IM/1 -> Demux4/1
  Servo_RIM/1 -> Gain_RIM/1
  Servo_PIM/1 -> Gain_PIM/1
  Servo_YIM/1 -> Gain_YIM/1
  Demux4/4 -> Servo_RIM/1
  Demux4/5 -> Servo_PIM/1
  Demux4/6 -> Servo_YIM/1
  Gain_act_RIM/1 -> Mux1/4
  Gain_act_PIM/1 -> Mux1/5
  Gain_act_YIM/1 -> Mux1/6
  OpLev_TM/1 -> Demux1/1
  IFO_TM/1 -> Servo_global_LIM/1
  Gain_LIM/1 -> Sum/1
  Servo_global_LIM/1 -> Gain_global_LIM/1
  Gain_PIM/1 -> Sum1/1
  Gain_YIM/1 -> Sum2/1
  Gain_global_LIM/1 -> Sum/2
  Servo_OpLev_PIM/1 -> Gain_OpLev_PIM/1
  Servo_OpLev_YIM/1 -> Gain_OpLev_YIM/1
  Gain_OpLev_PIM/1 -> Sum1/2
  Gain_OpLev_YIM/1 -> Sum2/2
  Sum/1 -> Sum3/1, Mux2/1
  Sum3/1 -> Gain_act_LIM/1
  Gain_TIM/1 -> Mux2/2, Sum4/1
  Sum4/1 -> Gain_act_TIM/1
  Gain_VIM/1 -> Mux2/3, Sum5/1
  Sum5/1 -> Gain_act_VIM/1
  Gain_RIM/1 -> Sum6/1, Mux2/4
  Sum6/1 -> Gain_act_RIM/1
  Sum1/1 -> Sum7/1, Mux2/5
  Sum7/1 -> Gain_act_PIM/1
  Sum2/1 -> Sum8/1, Mux2/6
  Sum8/1 -> Gain_act_YIM/1
  Demux2/1 -> Sum3/2
  Demux2/2 -> Sum4/2
  Demux2/3 -> Sum5/2
  Demux2/4 -> Sum6/2
  Demux2/5 -> Sum7/2
  Demux2/6 -> Sum8/2
  exc_IM/1 -> Demux2/1
  Mux2/1 -> fb_IM_mon/1
  Demux1/2 -> Servo_OpLev_PIM/1
  Demux1/3 -> Servo_OpLev_YIM/1
  Demux1/1 -> Terminator/1

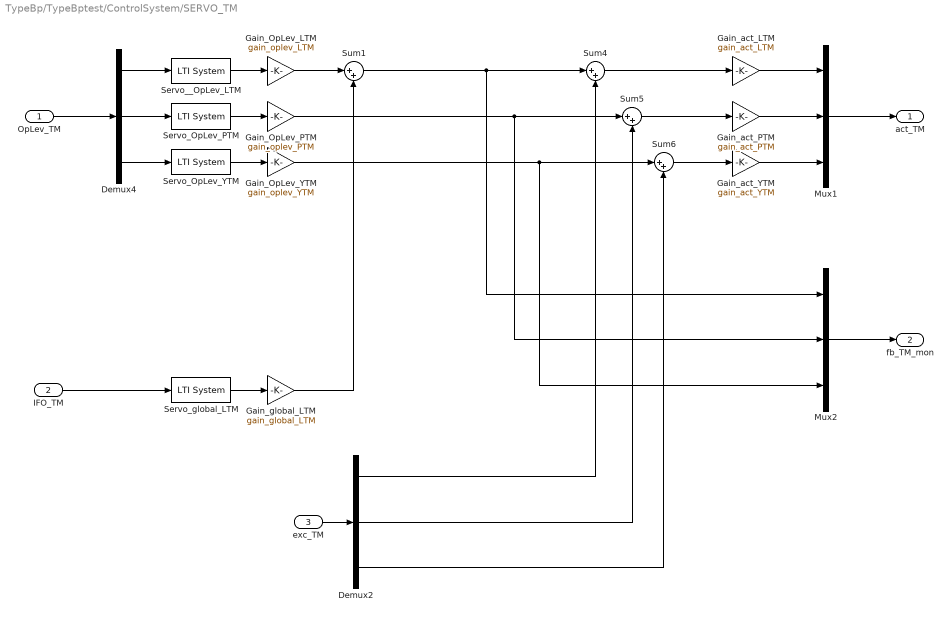
== system TypeBp/TypeBptest/ControlSystem/SERVO_TM ==
  OpLev_TM : Inport
  IFO_TM : Inport  Port=2
  exc_TM : Inport  Port=3
  Demux2 : Demux  Outputs=3
  Demux4 : Demux  Outputs=3
  Gain_OpLev_LTM : Gain  Gain=gain_oplev_LTM
  Gain_OpLev_PTM : Gain  Gain=gain_oplev_PTM
  Gain_OpLev_YTM : Gain  Gain=gain_oplev_YTM
  Gain_act_LTM : Gain  Gain=gain_act_LTM
  Gain_act_PTM : Gain  Gain=gain_act_PTM
  Gain_act_YTM : Gain  Gain=gain_act_YTM
  Gain_global_LTM : Gain  Gain=gain_global_LTM
  Mux1 : Mux  Inputs=3
  Mux2 : Mux  Inputs=3
  Servo_OpLev_PTM : cstblocks/LTI System  sys=servo_oplev_PTM  IC=[]
  Servo_OpLev_YTM : cstblocks/LTI System  sys=servo_oplev_YTM  IC=[]
  Servo__OpLev_LTM : cstblocks/LTI System  sys=servo_oplev_LTM  IC=[]
  Servo_global_LTM : cstblocks/LTI System  sys=servo_global_LTM  IC=[]
  Sum{1,4..6} (4 alike) : Sum  Inputs=|++
  act_TM : Outport
  fb_TM_mon : Outport  Port=2
  wires:
  Demux4/1 -> Servo__OpLev_LTM/1
  Demux4/2 -> Servo_OpLev_PTM/1
  Demux4/3 -> Servo_OpLev_YTM/1
  Servo__OpLev_LTM/1 -> Gain_OpLev_LTM/1
  Servo_OpLev_PTM/1 -> Gain_OpLev_PTM/1
  Servo_OpLev_YTM/1 -> Gain_OpLev_YTM/1
  OpLev_TM/1 -> Demux4/1
  Mux1/1 -> act_TM/1
  IFO_TM/1 -> Servo_global_LTM/1
  Servo_global_LTM/1 -> Gain_global_LTM/1
  Gain_OpLev_LTM/1 -> Sum1/1
  Gain_global_LTM/1 -> Sum1/2
  Gain_act_LTM/1 -> Mux1/1
  Gain_act_PTM/1 -> Mux1/2
  Gain_act_YTM/1 -> Mux1/3
  Sum1/1 -> Mux2/1, Sum4/1
  Sum4/1 -> Gain_act_LTM/1
  Gain_OpLev_PTM/1 -> Mux2/2, Sum5/1
  Sum5/1 -> Gain_act_PTM/1
  Gain_OpLev_YTM/1 -> Mux2/3, Sum6/1
  Sum6/1 -> Gain_act_YTM/1
  exc_TM/1 -> Demux2/1
  Demux2/1 -> Sum4/2
  Demux2/2 -> Sum5/2
  Demux2/3 -> Sum6/2
  Mux2/1 -> fb_TM_mon/1

== system TypeBp/TypeBptest/SuspensionSystem/M_IFO_TM ==
  disp_TM : Inport
  Add2 : Sum  Inputs=++++
  Demux4 : Demux  Outputs=6
  Gain1 : Gain  Gain=1/300
  Gain2 : Gain  Gain=1e-3
  Gain3 : Gain  Gain=1e-3
  Terminator1 : Terminator
  Terminator3 : Terminator
  sen_IFO : Outport
  wires:
  disp_TM/1 -> Demux4/1
  Demux4/4 -> Terminator3/1
  Demux4/3 -> Gain1/1
  Demux4/2 -> Terminator1/1
  Add2/1 -> sen_IFO/1
  Demux4/1 -> Add2/1
  Gain1/1 -> Add2/2
  Demux4/5 -> Gain2/1
  Gain3/1 -> Add2/4
  Gain2/1 -> Add2/3
  Demux4/6 -> Gain3/1

== system TypeBp/TypeBptest/SuspensionSystem/M_LVDT_GAS ==
  disp_GAS : Inport
  Add1 : Sum  Inputs=-+
  Add2 : Sum  Inputs=-+
  Demux4 : Demux  Outputs=3
  Mux3 : Mux  Inputs=2
  sen_LVDT : Outport
  wires:
  disp_GAS/1 -> Demux4/1
  Demux4/1 -> Add2/1
  Demux4/2 -> Add1/1, Add2/2
  Demux4/3 -> Add1/2
  Add2/1 -> Mux3/1
  Add1/1 -> Mux3/2
  Mux3/1 -> sen_LVDT/1

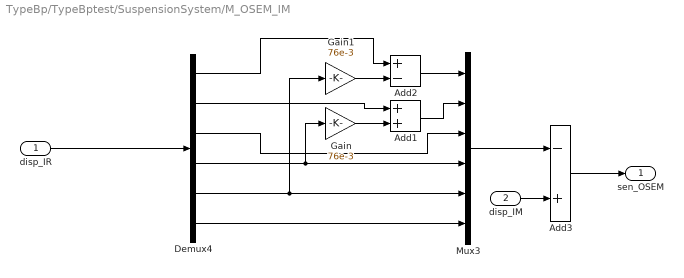
== system TypeBp/TypeBptest/SuspensionSystem/M_OSEM_IM ==
  disp_IR : Inport
  disp_IM : Inport  Port=2
  Add1 : Sum
  Add2 : Sum  Inputs=+-
  Add3 : Sum  Inputs=-+
  Demux4 : Demux  Outputs=6
  Gain : Gain  Gain=76e-3
  Gain1 : Gain  Gain=76e-3
  Mux3 : Mux  Inputs=6
  sen_OSEM : Outport
  wires:
  disp_IM/1 -> Add3/2
  disp_IR/1 -> Demux4/1
  Demux4/6 -> Mux3/6
  Mux3/1 -> Add3/1
  Add3/1 -> sen_OSEM/1
  Demux4/1 -> Add2/1
  Demux4/2 -> Add1/1
  Demux4/3 -> Mux3/3
  Demux4/4 -> Gain/1, Mux3/4
  Demux4/5 -> Gain1/1, Mux3/5
  Gain1/1 -> Add2/2
  Gain/1 -> Add1/2
  Add1/1 -> Mux3/2
  Add2/1 -> Mux3/1

== system TypeBp/TypeBptest/SuspensionSystem/M_OpLev_TM ==
  disp_TM : Inport
  Demux1 : Demux  Outputs=6
  Mux1 : Mux  Inputs=3
  Sens_Mat_OL : Constant  Value=Sens_Mat_OL  VectorParams1D=off
  TM_OpLev_coupling : Product  Multiplication=Matrix(*)
  Terminator4 : Terminator
  Terminator5 : Terminator
  Terminator6 : Terminator
  sen_OpLev : Outport
  wires:
  Demux1/5 -> Mux1/2
  Demux1/6 -> Mux1/3
  Demux1/4 -> Terminator6/1
  Demux1/3 -> Terminator5/1
  Demux1/2 -> Terminator4/1
  Demux1/1 -> Mux1/1
  Mux1/1 -> sen_OpLev/1
  TM_OpLev_coupling/1 -> Demux1/1
  Sens_Mat_OL/1 -> TM_OpLev_coupling/1
  disp_TM/1 -> TM_OpLev_coupling/2

== system TypeBp/TypeBptest/SuspensionSystem/M_SNS_BF ==
  disp_BR : Inport
  disp_F2 : Inport  Port=2
  Add2 : Sum  Inputs=-+
  sen_F2sensor : Outport
  wires:
  Add2/1 -> sen_F2sensor/1
  disp_BR/1 -> Add2/1
  disp_F2/1 -> Add2/2

== system TypeBp/TypeBptest/SuspensionSystem/M_act_F2 ==
  act_in : Inport
  Act_Mat_BF : Constant  Value=Act_Mat_BF  VectorParams1D=off
  Act_Mat_BR : Constant  Value=Act_Mat_BR  VectorParams1D=off
  BF_coupling : Product  Multiplication=Matrix(*)
  BR_coupling : Product  Multiplication=Matrix(*)
  Gain2 : Gain  Gain=-1
  act_out_BR : Outport
  act_out_F2 : Outport  Port=2
  wires:
  act_in/1 -> BF_coupling/2, Gain2/1
  Gain2/1 -> BR_coupling/2
  Act_Mat_BR/1 -> BR_coupling/1
  BR_coupling/1 -> act_out_BR/1
  Act_Mat_BF/1 -> BF_coupling/1
  BF_coupling/1 -> act_out_F2/1

== system TypeBp/TypeBptest/SuspensionSystem/M_act_GAS ==
  act_in : Inport
  Add1 : Sum  Inputs=+-
  Demux4 : Demux  Outputs=2
  Mux3 : Mux  Inputs=2
  act_out : Outport
  wires:
  act_in/1 -> Demux4/1
  Mux3/1 -> act_out/1
  Add1/1 -> Mux3/1
  Demux4/1 -> Add1/1
  Demux4/2 -> Add1/2, Mux3/2

== system TypeBp/TypeBptest/SuspensionSystem/M_act_IM ==
  act_in : Inport
  Act_Mat_IM : Constant  Value=Act_Mat_IM  VectorParams1D=off
  Act_Mat_IR : Constant  Value=Act_Mat_IR  VectorParams1D=off
  Gain2 : Gain  Gain=-1
  IM_coupling : Product  Multiplication=Matrix(*)
  IR_coupling : Product  Multiplication=Matrix(*)
  act_out_IR : Outport
  act_out_IM : Outport  Port=2
  wires:
  IR_coupling/1 -> act_out_IR/1
  Act_Mat_IR/1 -> IR_coupling/1
  act_in/1 -> IM_coupling/2, Gain2/1
  Act_Mat_IM/1 -> IM_coupling/1
  IM_coupling/1 -> act_out_IM/1
  Gain2/1 -> IR_coupling/2

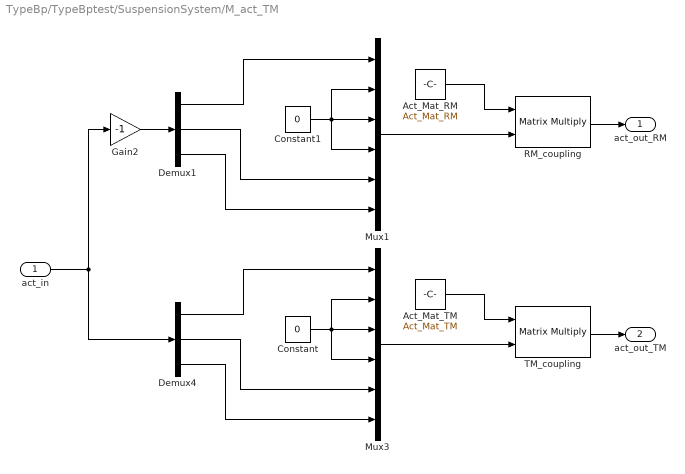
== system TypeBp/TypeBptest/SuspensionSystem/M_act_TM ==
  act_in : Inport
  Act_Mat_RM : Constant  Value=Act_Mat_RM  VectorParams1D=off
  Act_Mat_TM : Constant  Value=Act_Mat_TM  VectorParams1D=off
  Constant : Constant  Value=0
  Constant1 : Constant  Value=0
  Demux1 : Demux  Outputs=3
  Demux4 : Demux  Outputs=3
  Gain2 : Gain  Gain=-1
  Mux1 : Mux  Inputs=6
  Mux3 : Mux  Inputs=6
  RM_coupling : Product  Multiplication=Matrix(*)
  TM_coupling : Product  Multiplication=Matrix(*)
  act_out_RM : Outport
  act_out_TM : Outport  Port=2
  wires:
  Demux4/1 -> Mux3/1
  Demux4/2 -> Mux3/5
  Demux4/3 -> Mux3/6
  Constant/1 -> Mux3/4, Mux3/2, Mux3/3
  Mux3/1 -> TM_coupling/2
  Act_Mat_TM/1 -> TM_coupling/1
  TM_coupling/1 -> act_out_TM/1
  act_in/1 -> Demux4/1, Gain2/1
  Demux1/1 -> Mux1/1
  Demux1/2 -> Mux1/5
  Demux1/3 -> Mux1/6
  Constant1/1 -> Mux1/4, Mux1/2, Mux1/3
  Gain2/1 -> Demux1/1
  Mux1/1 -> RM_coupling/2
  Act_Mat_RM/1 -> RM_coupling/1
  RM_coupling/1 -> act_out_RM/1

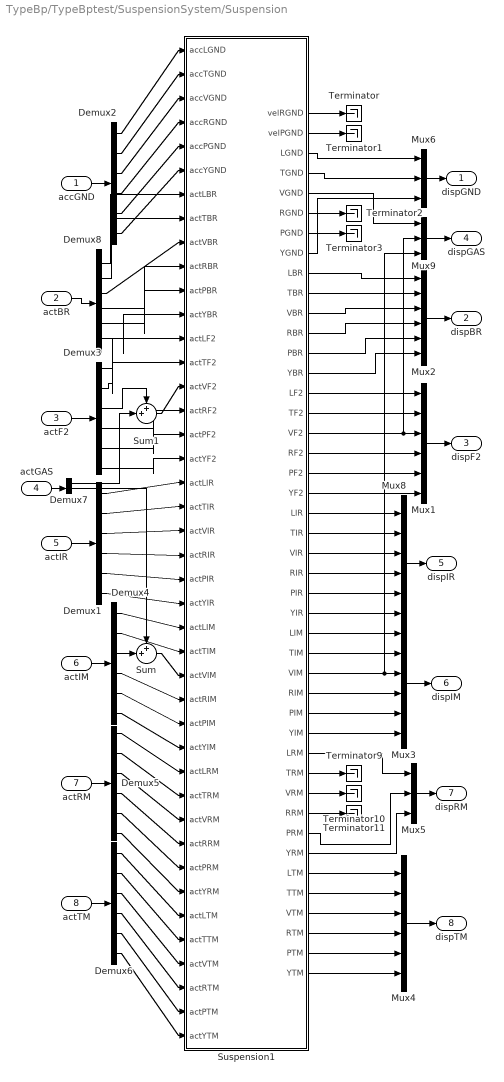
== system TypeBp/TypeBptest/SuspensionSystem/Suspension ==
  accGND : Inport
  actBR : Inport  Port=2
  actF2 : Inport  Port=3
  actGAS : Inport  Port=4
  actIR : Inport  Port=5
  actIM : Inport  Port=6
  actRM : Inport  Port=7
  actTM : Inport  Port=8
  Demux{1..6,8} (7 alike) : Demux  Outputs=6
  Demux7 : Demux  Outputs=2
  Mux{1..4,8} (5 alike) : Mux  Inputs=6
  Mux5 : Mux  Inputs=3
  Mux6 : Mux  Inputs=3
  Mux9 : Mux  Inputs=3
  Sum : Sum  Inputs=++|
  Sum1 : Sum  Inputs=++|
  Suspension1 : Subsystem
  Terminator{,1..3,9..11} (7 alike) : Terminator
  dispGND : Outport
  dispBR : Outport  Port=2
  dispF2 : Outport  Port=3
  dispGAS : Outport  Port=4
  dispIR : Outport  Port=5
  dispIM : Outport  Port=6
  dispRM : Outport  Port=7
  dispTM : Outport  Port=8
  wires:
  Mux3/1 -> dispIM/1
  Mux8/1 -> dispIR/1
  Mux4/1 -> dispTM/1
  accGND/1 -> Demux2/1
  actTM/1 -> Demux6/1
  actIR/1 -> Demux1/1
  actRM/1 -> Demux5/1
  actIM/1 -> Demux4/1
  Mux5/1 -> dispRM/1
  Demux6/5 -> Suspension1/41(actPTM)
  Demux2/5 -> Suspension1/5(accPGND)
  Demux6/3 -> Suspension1/39(actVTM)
  Demux2/6 -> Suspension1/6(accYGND)
  Demux2/1 -> Suspension1/1(accLGND)
  Demux2/3 -> Suspension1/3(accVGND)
  Demux6/4 -> Suspension1/40(actRTM)
  Demux2/2 -> Suspension1/2(accTGND)
  Demux2/4 -> Suspension1/4(accRGND)
  Demux6/2 -> Suspension1/38(actTTM)
  Demux6/6 -> Suspension1/42(actYTM)
  Suspension1/27(LIM) -> Mux3/1
  Suspension1/28(TIM) -> Mux3/2
  Suspension1/30(RIM) -> Mux3/4
  Suspension1/31(PIM) -> Mux3/5
  Suspension1/32(YIM) -> Mux3/6
  Suspension1/21(LIR) -> Mux8/1
  Suspension1/22(TIR) -> Mux8/2
  Suspension1/23(VIR) -> Mux8/3
  Suspension1/24(RIR) -> Mux8/4
  Suspension1/25(PIR) -> Mux8/5
  Suspension1/26(YIR) -> Mux8/6
  Mux6/1 -> dispGND/1
  actGAS/1 -> Demux7/1
  Demux7/2 -> Sum/1
  Suspension1/3(LGND) -> Mux6/1
  Suspension1/4(TGND) -> Mux6/2
  actF2/1 -> Demux3/1
  Demux6/1 -> Suspension1/37(actLTM)
  Demux4/4 -> Suspension1/28(actRIM)
  Demux1/1 -> Suspension1/19(actLIR)
  Demux1/2 -> Suspension1/20(actTIR)
  Demux1/3 -> Suspension1/21(actVIR)
  Demux1/4 -> Suspension1/22(actRIR)
  Demux1/5 -> Suspension1/23(actPIR)
  Demux1/6 -> Suspension1/24(actYIR)
  Demux4/1 -> Suspension1/25(actLIM)
  Demux4/2 -> Suspension1/26(actTIM)
  Sum/1 -> Suspension1/27(actVIM)
  Demux4/5 -> Suspension1/29(actPIM)
  Demux4/6 -> Suspension1/30(actYIM)
  Mux1/1 -> dispF2/1
  actBR/1 -> Demux8/1
  Demux8/1 -> Suspension1/7(actLBR)
  Demux8/2 -> Suspension1/8(actTBR)
  Demux3/1 -> Suspension1/13(actLF2)
  Demux3/2 -> Suspension1/14(actTF2)
  Demux4/3 -> Sum/2
  Demux7/1 -> Sum1/2
  Suspension1/8(YGND) -> Mux6/3
  Suspension1/1(velRGND) -> Terminator/1
  Suspension1/2(velPGND) -> Terminator1/1
  Suspension1/6(RGND) -> Terminator2/1
  Suspension1/7(PGND) -> Terminator3/1
  Mux2/1 -> dispBR/1
  Suspension1/9(LBR) -> Mux2/1
  Suspension1/10(TBR) -> Mux2/2
  Suspension1/15(LF2) -> Mux1/1
  Suspension1/16(TF2) -> Mux1/2
  Suspension1/29(VIM) -> Mux9/3, Mux3/3
  Mux9/1 -> dispGAS/1
  Suspension1/17(VF2) -> Mux9/2, Mux1/3
  Suspension1/5(VGND) -> Mux9/1
  Suspension1/33(LRM) -> Mux5/1
  Suspension1/37(PRM) -> Mux5/2
  Suspension1/38(YRM) -> Mux5/3
  Suspension1/34(TRM) -> Terminator9/1
  Suspension1/35(VRM) -> Terminator10/1
  Suspension1/36(RRM) -> Terminator11/1
  Suspension1/44(YTM) -> Mux4/6
  Suspension1/39(LTM) -> Mux4/1
  Suspension1/42(RTM) -> Mux4/4
  Suspension1/41(VTM) -> Mux4/3
  Suspension1/40(TTM) -> Mux4/2
  Suspension1/43(PTM) -> Mux4/5
  Demux8/3 -> Suspension1/9(actVBR)
  Demux8/4 -> Suspension1/10(actRBR)
  Demux8/5 -> Suspension1/11(actPBR)
  Demux8/6 -> Suspension1/12(actYBR)
  Demux3/3 -> Sum1/1
  Sum1/1 -> Suspension1/15(actVF2)
  Demux3/4 -> Suspension1/16(actRF2)
  Demux3/6 -> Suspension1/18(actYF2)
  Demux3/5 -> Suspension1/17(actPF2)
  Demux5/2 -> Suspension1/32(actTRM)
  Demux5/3 -> Suspension1/33(actVRM)
  Demux5/1 -> Suspension1/31(actLRM)
  Demux5/5 -> Suspension1/35(actPRM)
  Demux5/4 -> Suspension1/34(actRRM)
  Demux5/6 -> Suspension1/36(actYRM)
  Suspension1/11(VBR) -> Mux2/3
  Suspension1/12(RBR) -> Mux2/4
  Suspension1/13(PBR) -> Mux2/5
  Suspension1/14(YBR) -> Mux2/6
  Suspension1/18(RF2) -> Mux1/4
  Suspension1/19(PF2) -> Mux1/5
  Suspension1/20(YF2) -> Mux1/6

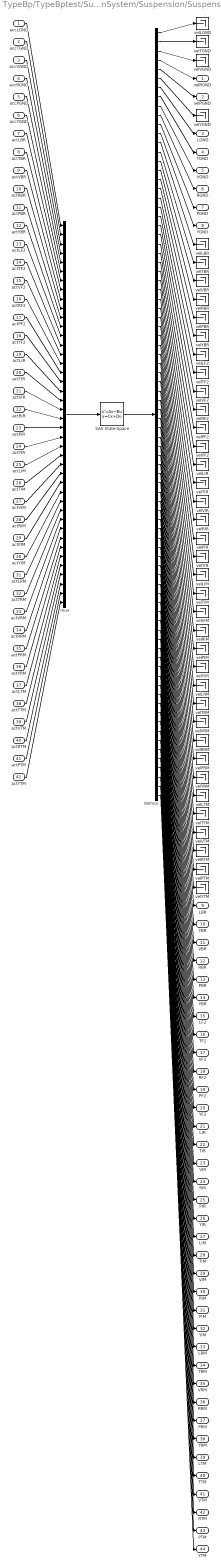
== system TypeBp/TypeBptest/SuspensionSystem/Suspension/Suspension1 ==
  accLGND : Inport
  accTGND : Inport  Port=2
  accVGND : Inport  Port=3
  accRGND : Inport  Port=4
  accPGND : Inport  Port=5
  accYGND : Inport  Port=6
  actLBR : Inport  Port=7
  actTBR : Inport  Port=8
  actVBR : Inport  Port=9
  actRBR : Inport  Port=10
  actPBR : Inport  Port=11
  actYBR : Inport  Port=12
  actLF2 : Inport  Port=13
  actTF2 : Inport  Port=14
  actVF2 : Inport  Port=15
  actRF2 : Inport  Port=16
  actPF2 : Inport  Port=17
  actYF2 : Inport  Port=18
  actLIR : Inport  Port=19
  actTIR : Inport  Port=20
  actVIR : Inport  Port=21
  actRIR : Inport  Port=22
  actPIR : Inport  Port=23
  actYIR : Inport  Port=24
  actLIM : Inport  Port=25
  actTIM : Inport  Port=26
  actVIM : Inport  Port=27
  actRIM : Inport  Port=28
  actPIM : Inport  Port=29
  actYIM : Inport  Port=30
  actLRM : Inport  Port=31
  actTRM : Inport  Port=32
  actVRM : Inport  Port=33
  actRRM : Inport  Port=34
  actPRM : Inport  Port=35
  actYRM : Inport  Port=36
  actLTM : Inport  Port=37
  actTTM : Inport  Port=38
  actVTM : Inport  Port=39
  actRTM : Inport  Port=40
  actPTM : Inport  Port=41
  actYTM : Inport  Port=42
  SAS State-Space : StateSpace  A=sys1.A  B=sys1.B  C=sys1.C  D=sys1.D  X0=0  ContinuousStateAttributes='SUS_SS_MODEL'
  demux : Demux  Outputs=84
  mux : Mux  Inputs=42
  velLBR : Terminator
  velLF2 : Terminator
  velLGND : Terminator
  velLIM : Terminator
  velLIR : Terminator
  velLRM : Terminator
  velLTM : Terminator
  velPBR : Terminator
  velPF2 : Terminator
  velPIM : Terminator
  velPIR : Terminator
  velPRM : Terminator
  velPTM : Terminator
  velRBR : Terminator
  velRF2 : Terminator
  velRIM : Terminator
  velRIR : Terminator
  velRRM : Terminator
  velRTM : Terminator
  velTBR : Terminator
  velTF2 : Terminator
  velTGND : Terminator
  velTIM : Terminator
  velTIR : Terminator
  velTRM : Terminator
  velTTM : Terminator
  velVBR : Terminator
  velVF2 : Terminator
  velVGND : Terminator
  velVIM : Terminator
  velVIR : Terminator
  velVRM : Terminator
  velVTM : Terminator
  velYBR : Terminator
  velYF2 : Terminator
  velYGND : Terminator
  velYIM : Terminator
  velYIR : Terminator
  velYRM : Terminator
  velYTM : Terminator
  velRGND : Outport
  velPGND : Outport  Port=2
  LGND : Outport  Port=3
  TGND : Outport  Port=4
  VGND : Outport  Port=5
  RGND : Outport  Port=6
  PGND : Outport  Port=7
  YGND : Outport  Port=8
  LBR : Outport  Port=9
  TBR : Outport  Port=10
  VBR : Outport  Port=11
  RBR : Outport  Port=12
  PBR : Outport  Port=13
  YBR : Outport  Port=14
  LF2 : Outport  Port=15
  TF2 : Outport  Port=16
  VF2 : Outport  Port=17
  RF2 : Outport  Port=18
  PF2 : Outport  Port=19
  YF2 : Outport  Port=20
  LIR : Outport  Port=21
  TIR : Outport  Port=22
  VIR : Outport  Port=23
  RIR : Outport  Port=24
  PIR : Outport  Port=25
  YIR : Outport  Port=26
  LIM : Outport  Port=27
  TIM : Outport  Port=28
  VIM : Outport  Port=29
  RIM : Outport  Port=30
  PIM : Outport  Port=31
  YIM : Outport  Port=32
  LRM : Outport  Port=33
  TRM : Outport  Port=34
  VRM : Outport  Port=35
  RRM : Outport  Port=36
  PRM : Outport  Port=37
  YRM : Outport  Port=38
  LTM : Outport  Port=39
  TTM : Outport  Port=40
  VTM : Outport  Port=41
  RTM : Outport  Port=42
  PTM : Outport  Port=43
  YTM : Outport  Port=44
  wires:
  mux/1 -> SAS State-Space/1
  SAS State-Space/1 -> demux/1
  accLGND/1 -> mux/1
  accTGND/1 -> mux/2
  accVGND/1 -> mux/3
  accRGND/1 -> mux/4
  accPGND/1 -> mux/5
  accYGND/1 -> mux/6
  actLBR/1 -> mux/7
  actTBR/1 -> mux/8
  actVBR/1 -> mux/9
  actRBR/1 -> mux/10
  actPBR/1 -> mux/11
  actYBR/1 -> mux/12
  actLF2/1 -> mux/13
  actTF2/1 -> mux/14
  actVF2/1 -> mux/15
  actRF2/1 -> mux/16
  actPF2/1 -> mux/17
  actYF2/1 -> mux/18
  actLIR/1 -> mux/19
  actTIR/1 -> mux/20
  actVIR/1 -> mux/21
  actRIR/1 -> mux/22
  actPIR/1 -> mux/23
  actYIR/1 -> mux/24
  actLIM/1 -> mux/25
  actTIM/1 -> mux/26
  actVIM/1 -> mux/27
  actRIM/1 -> mux/28
  actPIM/1 -> mux/29
  actYIM/1 -> mux/30
  actLRM/1 -> mux/31
  actTRM/1 -> mux/32
  actVRM/1 -> mux/33
  actRRM/1 -> mux/34
  actPRM/1 -> mux/35
  actYRM/1 -> mux/36
  actLTM/1 -> mux/37
  actTTM/1 -> mux/38
  actVTM/1 -> mux/39
  actRTM/1 -> mux/40
  actPTM/1 -> mux/41
  actYTM/1 -> mux/42
  demux/1 -> velLGND/1
  demux/2 -> velTGND/1
  demux/3 -> velVGND/1
  demux/4 -> velRGND/1
  demux/5 -> velPGND/1
  demux/6 -> velYGND/1
  demux/7 -> LGND/1
  demux/8 -> TGND/1
  demux/9 -> VGND/1
  demux/10 -> RGND/1
  demux/11 -> PGND/1
  demux/12 -> YGND/1
  demux/13 -> velLBR/1
  demux/14 -> velTBR/1
  demux/15 -> velVBR/1
  demux/16 -> velRBR/1
  demux/17 -> velPBR/1
  demux/18 -> velYBR/1
  demux/19 -> velLF2/1
  demux/20 -> velTF2/1
  demux/21 -> velVF2/1
  demux/22 -> velRF2/1
  demux/23 -> velPF2/1
  demux/24 -> velYF2/1
  demux/25 -> velLIR/1
  demux/26 -> velTIR/1
  demux/27 -> velVIR/1
  demux/28 -> velRIR/1
  demux/29 -> velPIR/1
  demux/30 -> velYIR/1
  demux/31 -> velLIM/1
  demux/32 -> velTIM/1
  demux/33 -> velVIM/1
  demux/34 -> velRIM/1
  demux/35 -> velPIM/1
  demux/36 -> velYIM/1
  demux/37 -> velLRM/1
  demux/38 -> velTRM/1
  demux/39 -> velVRM/1
  demux/40 -> velRRM/1
  demux/41 -> velPRM/1
  demux/42 -> velYRM/1
  demux/43 -> velLTM/1
  demux/44 -> velTTM/1
  demux/45 -> velVTM/1
  demux/46 -> velRTM/1
  demux/47 -> velPTM/1
  demux/48 -> velYTM/1
  demux/49 -> LBR/1
  demux/50 -> TBR/1
  demux/51 -> VBR/1
  demux/52 -> RBR/1
  demux/53 -> PBR/1
  demux/54 -> YBR/1
  demux/55 -> LF2/1
  demux/56 -> TF2/1
  demux/57 -> VF2/1
  demux/58 -> RF2/1
  demux/59 -> PF2/1
  demux/60 -> YF2/1
  demux/61 -> LIR/1
  demux/62 -> TIR/1
  demux/63 -> VIR/1
  demux/64 -> RIR/1
  demux/65 -> PIR/1
  demux/66 -> YIR/1
  demux/67 -> LIM/1
  demux/68 -> TIM/1
  demux/69 -> VIM/1
  demux/70 -> RIM/1
  demux/71 -> PIM/1
  demux/72 -> YIM/1
  demux/73 -> LRM/1
  demux/74 -> TRM/1
  demux/75 -> VRM/1
  demux/76 -> RRM/1
  demux/77 -> PRM/1
  demux/78 -> YRM/1
  demux/79 -> LTM/1
  demux/80 -> TTM/1
  demux/81 -> VTM/1
  demux/82 -> RTM/1
  demux/83 -> PTM/1
  demux/84 -> YTM/1
